simulink model "hydcyl"  (Simulink 6.0)
settings: Solver=ode45  SolverMode=SingleTasking  StartTime=0  StopTime=0.1  RelTol=1e-4  AbsTol=1e-6
PreLoadFcn:
  | load newhcd
undefined symbols (not defined in the file or in its folder): C2, K, Qmax
libraries: hydlib x2
settings Model: CovMetricSettings=d  Creator=The MathWorks Inc.  LastModifiedBy=batserve  ExtModeTrigMode=oneshot  ExtModeArmWhenConnect=off  ExtModeAutoUpdateStatusClock=off
settings DataIOCC: LimitDataPoints=off  SaveState=on
settings OptimizationCC: BlockReduction=off  BooleanDataType=off
settings DebuggingCC: AlgebraicLoopMsg=none  CheckExecutionContextPreStartOutputMsg=on  CheckExecutionContextRuntimeOutputMsg=on  SolverPrmCheckMsg=none  IntegerOverflowMsg=none
settings HardwareCC: TargetUnknown=on

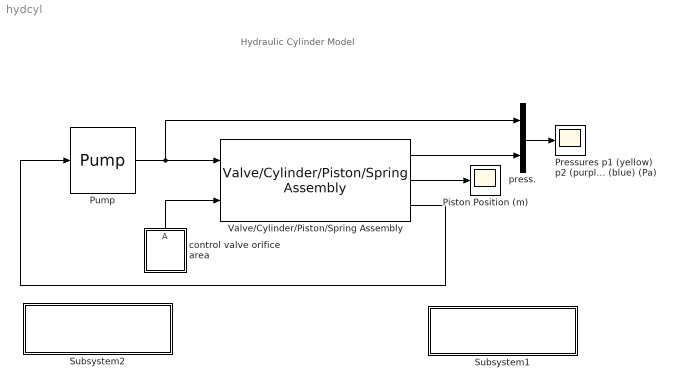
== system hydcyl ==
  note: Hydraulic Cylinder Model
  Piston Position (m) : Scope
      settings: TickLabels=on  TimeRange=0.1  YMin=0  YMax=0.04  DataFormat=Array
  Pressures p1 (yellow) p2 (purple) p3 (blue) (Pa) : Scope
      settings: TickLabels=on  TimeRange=0.1  YMin=0  YMax=2e+06  DataFormat=Array
  Pump : hydlib/Pump  t="[0        .04     .04     .05    .05     .1]"  Qpump=Qmax*[1 1 0 0 1 1]  p10=Qmax/C2*2  C2=C2
  Subsystem1 : Subsystem  PropExecContextAcrossSSBoundary=on
      settings: OpenFcn=hydcyl4
      mask Type: Button
      mask Display: disp('Double click to see\na 4 cylinder model.')
  Subsystem2 : Subsystem  PropExecContextAcrossSSBoundary=on
      settings: OpenFcn=sim(get_param(0,'CurrentSystem'),0.1)
      mask Type: Button
      mask Display: disp('Double click to run the \nSimulation for 0.1 seconds')
  Valve/Cylinder/Piston/Spring Assembly : hydlib/Valve//Cylinder//Piston//Spring Assembly  K=K  C1=C1  Ac=Ac  Cd=Cd  rho=rho  V30=V30  beta=Beta
  control valve orifice area : Subsystem  Orientation=up  PropExecContextAcrossSSBoundary=on
      mask Type: Ramp
      mask Display: plot(0,0,100,100,[98,0],[96,0])
  press. : Mux  Inputs=2
  wires:
  control valve orifice area/1(A) -> Valve/Cylinder/Piston/Spring Assembly/2
  Pump/1 -> Valve/Cylinder/Piston/Spring Assembly/1, press./1
  press./1 -> Pressures p1 (yellow) p2 (purple) p3 (blue) (Pa)/1
  Valve/Cylinder/Piston/Spring Assembly/2 -> Piston Position (m)/1
  Valve/Cylinder/Piston/Spring Assembly/1 -> press./2
  Valve/Cylinder/Piston/Spring Assembly/3 -> Pump/1

== system hydcyl/Subsystem1 ==

== system hydcyl/Subsystem2 ==

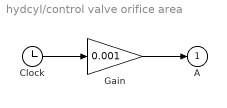
== system hydcyl/control valve orifice area ==
  Clock : Clock
      settings: Decimation=10
  Gain : Gain  Gain=0.001  SaturateOnIntegerOverflow=on
  A : Outport  InitialOutput=0
  wires:
  Gain/1 -> A/1
  Clock/1 -> Gain/1
